simulink model "Case3_Sim"  (R2020b)
settings: Solver=FixedStepAuto  StartTime=0.0  StopTime=10  FixedStep=Ts  RelTol=1e-3
values from neighbouring files (symbols this model uses):
  Cf = 0.02    [Case3_SimPara.m]
  Lc = 1e-9    (= 1e-09)    [Case3_SimPara.m]
  Lf = 0.05    [Case3_SimPara.m]
  Sbase = 1    [Case3_SimPara.m]
  Ts = 1/Fs    (= 0.0001)    [Case3_SimPara.m]
  Vbase = 1    [Case3_SimPara.m]
  w_i = 250*2*pi    (= 1570.79632679)    [Case3_SimPara.m]
  w_pll = 15*2*pi    (= 94.2477796077)    [Case3_SimPara.m]
  w_tau = 1e3*2*pi    (= 6283.18530718)    [Case3_SimPara.m]
  Wbase = 2*pi*50    (= 314.159265359)    [Case3_SimPara.m]
  Ybase = 1/Zbase    (= 1)    [Case3_SimPara.m]
  Zbase = Vbase/Ibase    (= 1)    [Case3_SimPara.m]
undefined symbols (not defined in the file or in its folder): DiscIntNeverNeededParam, initial, m
libraries: SimplexPS x25, powerlib x21
settings Model: Creator=admin_user  LastModifiedBy=admin_user
settings DataIOCC: ReturnWorkspaceOutputs=off

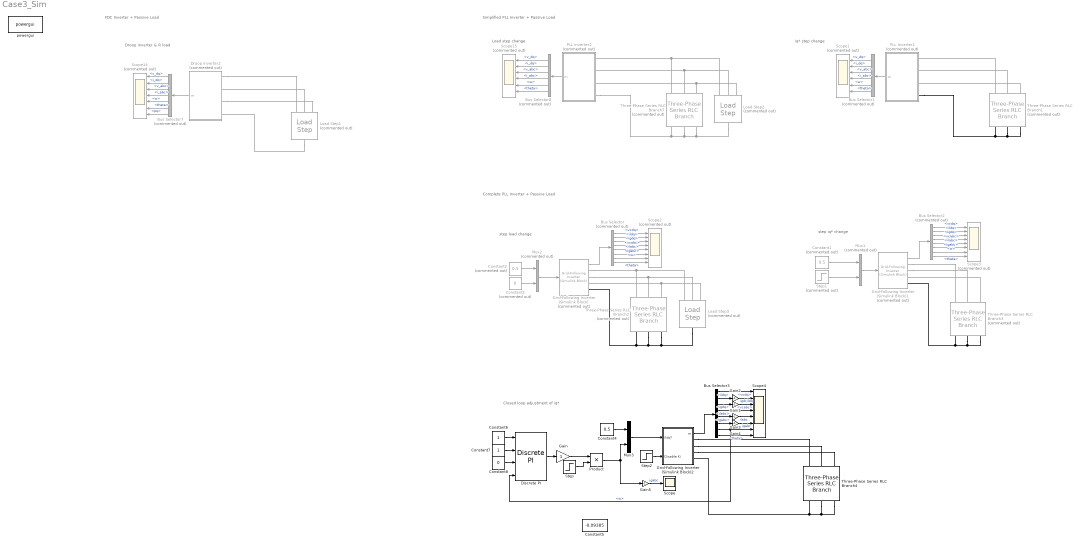
== system Case3_Sim ==
  note: step load change
  note: iq* step change
  note: Load step change
  note: FDC Inverter + Passive Load
  note: Droop inverter & R load
  note: Simplified PLL Inverter + Passive Load
  note: Complete PLL Inverter + Passive Load
  note: step iq* change
  note: Closed loop adjustment of iq*
  Bus Selector : BusSelector  Commented=on  OutputSignals=vcdq,ildq,igdq,vcabc,ilabc,igabc,w,theta
  Bus Selector1 : BusSelector  Commented=on  OutputSignals=v_dq,i_dq,v_abc,i_abc,w,theta
  Bus Selector2 : BusSelector  Commented=on  OutputSignals=vcdq,ildq,igdq,vcabc,ilabc,igabc,w,theta
  Bus Selector3 : BusSelector  OutputSignals=vcdq,ildq,igdq,vcabc,ilabc,igabc,w,theta
  Bus Selector7 : BusSelector  Commented=on  OutputSignals=v_dq,i_dq,v_abc,i_abc,w,theta,pq
  Bus Selector8 : BusSelector  Commented=on  OutputSignals=v_dq,i_dq,v_abc,i_abc,w,theta
  Constant1 : Constant  Commented=on  Value=0.5
  Constant2 : Constant  Commented=on  Value=0.5
  Constant3 : Constant  Commented=on  Value=0
  Constant4 : Constant  Value=0.5
  Constant5 : Constant  Value=-0.09385
  Constant6 : Constant
  Constant7 : Constant
  Constant8 : Constant  Value=0
  Discrete PI : SimplexPS/Discrete PI  Kp=0.5*2*pi/5  Ki=(0.5*2*pi)^2/4/5  xmax=inf  xmin=-inf  Ts=Ts
      settings: SourceProductName=Simplex Power Systems
  Droop Inverter2 : Subsystem  Commented=on
  Gain : Gain
  Gain{1..5} (5 alike) : Gain  Gain=-1
  Grid-Following Inverter (Simulink Block) : SimplexPS/Grid-Following Inverter (Simulink Block)  Commented=on  Ts=Ts  Sbase=Sbase  Vbase=Vbase  Wbase=Wbase  w_i=w_i  w_pll=w_pll  w_tau=w_tau  Lf=Lf  Cf=Cf  Lc=Lc
      link override ControllerAC/Current Controller: Ki=w_i*Lf*w_i/4
      link override Current Controller: Kcd=0
      link override LC Filter: Rd=1e-9
      settings: SourceProductName=Simplex Power Systems
  Grid-Following Inverter (Simulink Block)1 : SimplexPS/Grid-Following Inverter (Simulink Block)  Commented=on  Ts=Ts  Sbase=Sbase  Vbase=Vbase  Wbase=Wbase  w_i=w_i  w_pll=w_pll  w_tau=w_tau  Lf=Lf  Cf=Cf  Lc=Lc
      link override ControllerAC/Current Controller: Ki=w_i*Lf*w_i/4
      link override Current Controller: Kcd=0
      link override LC Filter: Rd=1e-9
      settings: SourceProductName=Simplex Power Systems
  Grid-Following Inverter (Simulink Block)2 : Subsystem  AncestorBlock=|
      | SimplexPS/Grid-Following Inverter
      | (Simulink Block)
  Load Step1 : SimplexPS/Load Step  Commented=on  t0=1  R=2*Zbase  Reverse=0
      settings: SourceProductName=Simplex Power Systems
  Load Step2 : SimplexPS/Load Step  Commented=on  t0=1  R=Zbase  Reverse=0
      settings: SourceProductName=Simplex Power Systems
  Load Step3 : SimplexPS/Load Step  Commented=on  t0=1  R=Zbase  Reverse=0
      settings: SourceProductName=Simplex Power Systems
  Mux1 : Mux  Commented=on  Inputs=2
  Mux2 : Mux  Commented=on  Inputs=2
  Mux3 : Mux  Inputs=2
  PLL Inverter1 : Subsystem  Commented=on
  PLL Inverter2 : Subsystem  Commented=on
  Product : Product
  Scope : Scope
  Scope1 : Scope  Commented=on  NumInputPorts=6
  Scope14 : Scope  Commented=on  NumInputPorts=7
  Scope15 : Scope  Commented=on  NumInputPorts=6
  Scope2 : Scope  Commented=on  NumInputPorts=8
  Scope3 : Scope  Commented=on  NumInputPorts=8
  Scope4 : Scope  NumInputPorts=8
  Step : Step  Time=9  Before=1  After=0  SampleTime=0
  Step1 : Step  Commented=on  After=0.1  SampleTime=0
  Step2 : Step  Time=9.4  Before=1  After=0  SampleTime=0
  Three-Phase Series RLC Branch{1..3,7} (4 alike) : powerlib/Elements/Three-Phase Series RLC Branch  Commented=on  LConnTagsString=A|B|C  RConnTagsString=A|B|C  BranchType=R  Resistance=Zbase  Inductance=0.3*Zbase/Wbase  Capacitance=1/Wbase  Measurements=None
  Three-Phase Series RLC Branch4 : powerlib/Elements/Three-Phase Series RLC Branch  LConnTagsString=A|B|C  RConnTagsString=A|B|C  BranchType=RL  Resistance=Zbase  Inductance=0.2*Zbase/Wbase  Capacitance=1/Wbase  Measurements=None
  powergui : powerlib/powergui  Priority=1  SimulationMode=Discrete  SampleTime=Ts  frequency=60  Iterations=50  frequencyindice=0  Pbase=100e6  ErrMax=1e-4  UnitsV=kV  UnitsW=MW  buscounter=0  FunctionMessages=off  echomessages=off  EnableUseOfTLC=off  CurrentSourceSwitches=off  DisableSnubberDevices=off  DisableRonSwitches=off  DisableVfSwitches=off  DisplayEquations=off  AutomaticDiscreteSolvers=off  SolverType=Tustin/Backward Euler (TBE)  Interpol=off  ExternalGateDelay=off  methode=off  Ts=100  x0status=blocks  SPID=on  SwTol=0  HookPort=off  NonlinearTolerance=1e-4  nMaxIteration=100  ContinueOnMaxIteration=off  RestoreLinks=warning  ResistiveCurrentMeasurement=off  Frange=[0:2:500]  Ylog=off  Xlog=on  ShowGrid=off  save=off  variable=ZData  structure=0  ZoomFFT=off  StartTime=0.0  cycles=1  DisplayStyle=1  fundamental=60  FreqAxis=off  MaxFrequency=1000  frequencyindicesteady=1  RmsSteady=1  display=off
  wires:
  Bus Selector7/3 -> Scope14/3  "<v_abc>"
  Bus Selector7/6 -> Scope14/6  "<theta>"
  Bus Selector7/2 -> Scope14/2  "<i_dq>"
  Bus Selector7/1 -> Scope14/1  "<v_dq>"
  Droop Inverter2/1(m) -> Bus Selector7/1
  Bus Selector7/7 -> Scope14/7  "<pq>"
  Bus Selector7/5 -> Scope14/5  "<w>"
  Bus Selector7/4 -> Scope14/4  "<i_abc>"
  PLL Inverter2/1(m) -> Bus Selector8/1
  Bus Selector8/2 -> Scope15/2  "<i_dq>"
  Bus Selector8/1 -> Scope15/1  "<v_dq>"
  Bus Selector8/4 -> Scope15/4  "<i_abc>"
  Bus Selector8/3 -> Scope15/3  "<v_abc>"
  Bus Selector8/6 -> Scope15/6  "<theta>"
  Bus Selector8/5 -> Scope15/5  "<w>"
  PLL Inverter1/1(m) -> Bus Selector1/1
  Bus Selector1/6 -> Scope1/6  "<theta>"
  Bus Selector1/3 -> Scope1/3  "<v_abc>"
  Bus Selector1/2 -> Scope1/2  "<i_dq>"
  Bus Selector1/1 -> Scope1/1  "<v_dq>"
  Bus Selector1/5 -> Scope1/5  "<w>"
  Bus Selector1/4 -> Scope1/4  "<i_abc>"
  Grid-Following Inverter (Simulink Block)/1 -> Bus Selector/1
  Bus Selector/1 -> Scope2/1  "<vcdq>"
  Bus Selector/2 -> Scope2/2  "<ildq>"
  Bus Selector/3 -> Scope2/3  "<igdq>"
  Bus Selector/4 -> Scope2/4  "<vcabc>"
  Bus Selector/5 -> Scope2/5  "<ilabc>"
  Bus Selector/6 -> Scope2/6  "<igabc>"
  Bus Selector/7 -> Scope2/7  "<w>"
  Bus Selector/8 -> Scope2/8  "<theta>"
  Grid-Following Inverter (Simulink Block)1/1 -> Bus Selector2/1
  Step1/1 -> Mux1/2
  Constant1/1 -> Mux1/1
  Mux1/1 -> Grid-Following Inverter (Simulink Block)1/1
  Bus Selector2/8 -> Scope3/8  "<theta>"
  Bus Selector2/5 -> Scope3/5  "<ilabc>"
  Bus Selector2/7 -> Scope3/7  "<w>"
  Bus Selector2/3 -> Scope3/3  "<igdq>"
  Bus Selector2/4 -> Scope3/4  "<vcabc>"
  Bus Selector2/6 -> Scope3/6  "<igabc>"
  Bus Selector2/1 -> Scope3/1  "<vcdq>"
  Bus Selector2/2 -> Scope3/2  "<ildq>"
  Mux2/1 -> Grid-Following Inverter (Simulink Block)/1
  Constant2/1 -> Mux2/1
  Constant3/1 -> Mux2/2
  Grid-Following Inverter (Simulink Block)2/1(m) -> Bus Selector3/1
  Mux3/1 -> Grid-Following Inverter (Simulink Block)2/1(ildq*)
  Constant4/1 -> Mux3/1
  Bus Selector3/8 -> Scope4/8  "<theta>"
  Bus Selector3/7 -> Discrete PI/4, Scope4/7  "<w>"
  Bus Selector3/4 -> Scope4/4  "<vcabc>"
  Bus Selector3/1 -> Scope4/1  "<vcdq>"
  Constant6/1 -> Discrete PI/1
  Constant7/1 -> Discrete PI/2
  Constant8/1 -> Discrete PI/3
  Product/1 -> Gain5/1, Mux3/2
  Discrete PI/1 -> Gain/1
  Gain/1 -> Product/1
  Step/1 -> Product/2
  Step2/1 -> Grid-Following Inverter (Simulink Block)2/2(Disable Ki)
  Bus Selector3/3 -> Gain1/1  "<igdq>"
  Gain1/1 -> Scope4/3  "igdq"
  Bus Selector3/2 -> Gain2/1  "<ildq>"
  Gain2/1 -> Scope4/2  "ildq"
  Gain3/1 -> Scope4/5  "ilabc"
  Bus Selector3/5 -> Gain3/1  "<ilabc>"
  Gain4/1 -> Scope4/6  "igabc"
  Bus Selector3/6 -> Gain4/1  "<igabc>"
  Gain5/1 -> Scope/1  "igabc"
  connections:
  Droop Inverter2/LConn1 -- Load Step1/LConn1
  Load Step1/LConn2 -- Droop Inverter2/LConn2
  Droop Inverter2/LConn3 -- Load Step1/LConn3
  Load Step1/RConn1 -- Droop Inverter2/LConn4
  Three-Phase Series RLC Branch7/RConn1 -- Load Step2/LConn1 -- PLL Inverter2/LConn1
  Three-Phase Series RLC Branch7/RConn2 -- Load Step2/LConn2 -- PLL Inverter2/LConn2
  Three-Phase Series RLC Branch7/RConn3 -- Load Step2/LConn3 -- PLL Inverter2/LConn3
  PLL Inverter2/LConn4 -- Load Step2/RConn1 -- Three-Phase Series RLC Branch7/LConn3 -- Three-Phase Series RLC Branch7/LConn2 -- Three-Phase Series RLC Branch7/LConn1
  Three-Phase Series RLC Branch1/RConn2 -- PLL Inverter1/LConn2
  Three-Phase Series RLC Branch1/RConn3 -- PLL Inverter1/LConn3
  Three-Phase Series RLC Branch1/LConn1 -- PLL Inverter1/LConn4 -- Three-Phase Series RLC Branch1/LConn3 -- Three-Phase Series RLC Branch1/LConn2
  Three-Phase Series RLC Branch1/RConn1 -- PLL Inverter1/LConn1
  Three-Phase Series RLC Branch2/RConn2 -- Load Step3/LConn2 -- Grid-Following Inverter (Simulink Block)/RConn2
  Three-Phase Series RLC Branch2/RConn3 -- Load Step3/LConn3 -- Grid-Following Inverter (Simulink Block)/RConn3
  Three-Phase Series RLC Branch2/LConn1 -- Load Step3/RConn1 -- Three-Phase Series RLC Branch2/LConn3 -- Three-Phase Series RLC Branch2/LConn2 -- Grid-Following Inverter (Simulink Block)/RConn4
  Load Step3/LConn1 -- Grid-Following Inverter (Simulink Block)/RConn1 -- Three-Phase Series RLC Branch2/RConn1
  Three-Phase Series RLC Branch3/LConn1 -- Grid-Following Inverter (Simulink Block)1/RConn4 -- Three-Phase Series RLC Branch3/LConn3 -- Three-Phase Series RLC Branch3/LConn2
  Three-Phase Series RLC Branch3/RConn3 -- Grid-Following Inverter (Simulink Block)1/RConn3
  Grid-Following Inverter (Simulink Block)1/RConn2 -- Three-Phase Series RLC Branch3/RConn2
  Grid-Following Inverter (Simulink Block)1/RConn1 -- Three-Phase Series RLC Branch3/RConn1
  Three-Phase Series RLC Branch4/LConn1 -- Grid-Following Inverter (Simulink Block)2/RConn4 -- Three-Phase Series RLC Branch4/LConn3 -- Three-Phase Series RLC Branch4/LConn2
  Grid-Following Inverter (Simulink Block)2/RConn2 -- Three-Phase Series RLC Branch4/RConn2
  Grid-Following Inverter (Simulink Block)2/RConn1 -- Three-Phase Series RLC Branch4/RConn1
  Grid-Following Inverter (Simulink Block)2/RConn3 -- Three-Phase Series RLC Branch4/RConn3

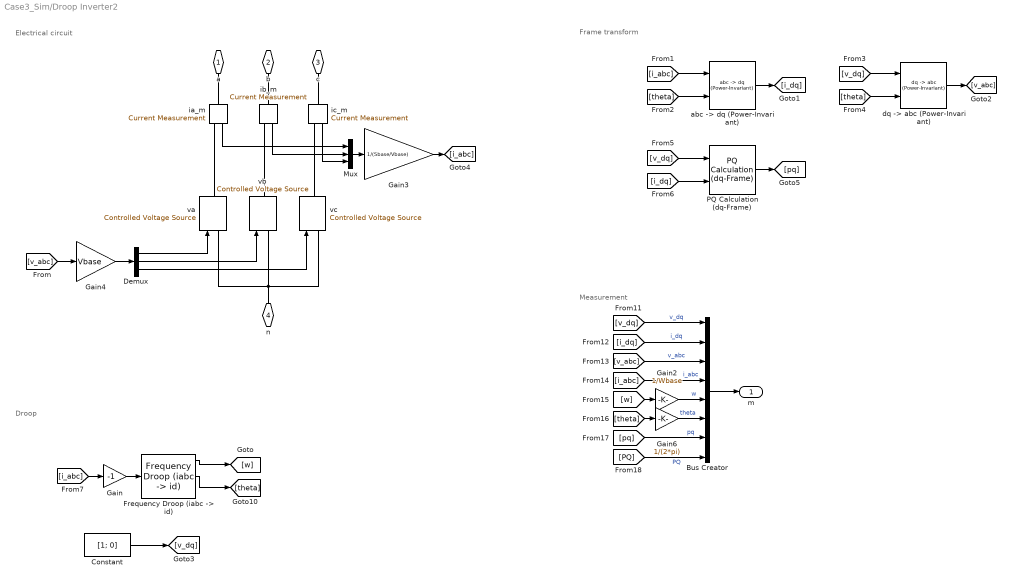
== system Case3_Sim/Droop Inverter2 ==
  note: Measurement
  note: Droop
  note: Frame transform
  note: Electrical circuit
  Bus Creator : BusCreator  Inputs=8
  Constant : Constant  Value=[1; 0]
  Demux : Demux  Outputs=3
  "Frequency Droop (iabc -> id)" : SimplexPS/Frequency Droop (iabc -> id)  Ts=Ts  Sbase=Sbase  Vbase=Vbase  Wbase=Wbase  m=m  w_tau=w_droop  theta0=0  i0=0  w0=1
      settings: SourceProductName=Simplex Power Systems
  Gain : Gain  Gain=-1
  Gain2 : Gain  Gain=1/Wbase
  Gain3 : Gain  Gain=1/(Sbase/Vbase)
  Gain4 : Gain  Gain=Vbase
  Gain6 : Gain  Gain=1/(2*pi)
  Mux : Mux  Inputs=3
  PQ Calculation (dq-Frame) : SimplexPS/PQ Calculation (dq-Frame)  SystemSampleTime=-1  VariantActivationTime=update diagram  Latency=0  AutoFrameSizeCalculation=off
      settings: SourceProductName=Simplex Power Systems
  "abc -> dq (Power-Invariant)" : SimplexPS/abc -> dq (Power-Invariant)  SystemSampleTime=-1  VariantActivationTime=update diagram  Latency=0  AutoFrameSizeCalculation=off
      settings: SourceProductName=Simplex Power Systems
  "dq -> abc (Power-Invariant)" : SimplexPS/dq -> abc (Power-Invariant)  SystemSampleTime=-1  VariantActivationTime=update diagram  Latency=0  AutoFrameSizeCalculation=off
      settings: SourceProductName=Simplex Power Systems
  ia_m : powerlib/Measurements/Current Measurement  PhasorSimulation=off  OutputType=Complex  PSBequivalent=0
  ib_m : powerlib/Measurements/Current Measurement  PhasorSimulation=off  OutputType=Complex  PSBequivalent=0
  ic_m : powerlib/Measurements/Current Measurement  PhasorSimulation=off  OutputType=Complex  PSBequivalent=0
  va : powerlib/Electrical Sources/Controlled Voltage Source  Initialize=on  Source_Type=AC  Amplitude=0  Phase=0  Frequency=0  Measurements=None
  vb : powerlib/Electrical Sources/Controlled Voltage Source  Initialize=on  Source_Type=AC  Amplitude=0  Phase=0  Frequency=0  Measurements=None
  vc : powerlib/Electrical Sources/Controlled Voltage Source  Initialize=on  Source_Type=AC  Amplitude=0  Phase=0  Frequency=0  Measurements=None
  a : PMIOPort  Side=Left
  b : PMIOPort  Port=2  Side=Left
  c : PMIOPort  Port=3  Side=Left
  n : PMIOPort  Port=4  Side=Left
  m : Outport
  wires:
  ic_m/1 -> Mux/3
  ia_m/1 -> Mux/1
  ib_m/1 -> Mux/2
  Demux/1 -> va/1
  Demux/2 -> vb/1
  Demux/3 -> vc/1
  [i_abc] -> "abc -> dq (Power-Invariant)"/1
  [theta] -> "abc -> dq (Power-Invariant)"/2
  "abc -> dq (Power-Invariant)"/1 -> [i_dq]
  [v_dq] -> "dq -> abc (Power-Invariant)"/1
  [theta] -> "dq -> abc (Power-Invariant)"/2
  "dq -> abc (Power-Invariant)"/1 -> [v_abc]
  [v_dq] -> Bus Creator/1  "v_dq"
  [v_abc] -> Bus Creator/3  "v_abc"
  [i_abc] -> Bus Creator/4  "i_abc"
  [pq] -> Bus Creator/7  "pq"
  [PQ] -> Bus Creator/8  "PQ"
  Bus Creator/1 -> m/1
  [w] -> Gain2/1
  Gain2/1 -> Bus Creator/5  "w"
  Mux/1 -> Gain3/1
  Gain3/1 -> [i_abc]
  [v_abc] -> Gain4/1
  Gain4/1 -> Demux/1
  [theta] -> Gain6/1
  Gain6/1 -> Bus Creator/6  "theta"
  "Frequency Droop (iabc -> id)"/2 -> [theta]
  [i_abc] -> Gain/1
  "Frequency Droop (iabc -> id)"/1 -> [w]
  Constant/1 -> [v_dq]
  [i_dq] -> Bus Creator/2  "i_dq"
  [v_dq] -> PQ Calculation (dq-Frame)/1
  [i_dq] -> PQ Calculation (dq-Frame)/2
  PQ Calculation (dq-Frame)/1 -> [pq]
  Gain/1 -> "Frequency Droop (iabc -> id)"/1
  connections:
  ia_m/RConn1 -- va/RConn1
  ia_m/LConn1 -- a/RConn1
  ib_m/RConn1 -- vb/RConn1
  ic_m/RConn1 -- vc/RConn1
  va/LConn1 -- vb/LConn1 -- vc/LConn1 -- n/RConn1
  ib_m/LConn1 -- b/RConn1
  ic_m/LConn1 -- c/RConn1

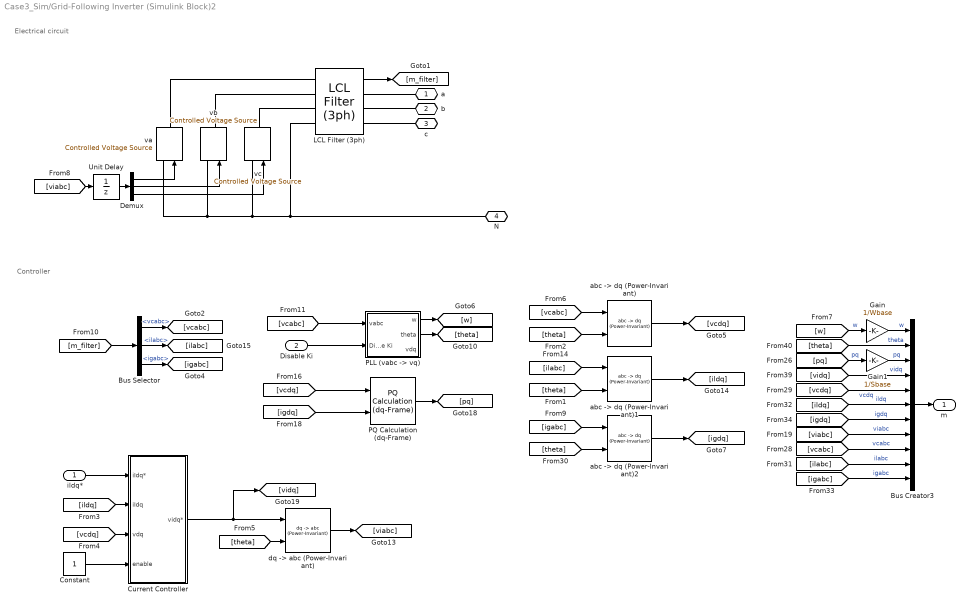
== system Case3_Sim/Grid-Following Inverter (Simulink Block)2 ==
  note: Electrical circuit
  note: Controller
  ildq* : Inport
  Disable Ki : Inport  Port=2
  Bus Creator3 : BusCreator  Inputs=11
  Bus Selector : BusSelector  OutputSignals=vcabc,ilabc,igabc
  Constant : Constant
  Current Controller : Subsystem  mask{Ts=Ts, Wbase=Wbase, Lf=Lf*Zbase/Wbase, Kg=0, Kp=w_i*Lf*Zbase/Wbase, Ki=w_i*w_i/4*Lf*Zbase/Wbase, vdmax=inf, vqmax=inf, Kcd=0}
      mask prompts: Ts "Sampling Time (s)"; Wbase "Base Angular Frequency (rad/s)"; Lf "Inductance"; Kg "Estimator Gain"; Kp "Proportional Gain"; Ki "Integral Gain"; vdmax "Voltage D Limit"; vqmax "Voltage Q Limit"; Kcd "Cross Decoupling Gain"
  Demux : Demux  Outputs=3
  Gain : Gain  Gain=1/Wbase
  Gain1 : Gain  Gain=1/Sbase
  LCL Filter (3ph) : SimplexPS/LCL Filter (3ph)  Lf=Lf*Zbase/Wbase  Rf=Lf/5  Lc=Lc*Zbase/Wbase  Rc=Lc/5  Cf=Cf*Ybase/Wbase  Rd=1e-20
      settings: SourceProductName=Simplex Power System
  "PLL (vabc -> vq)" : Subsystem  AncestorBlock=|  mask{Ts=Ts, Vbase=Vbase, Wbase=Wbase, w_pll=w_pll, w_tau=w_tau, theta0=0}
      | SimplexPS/PLL
      | (vabc -> vq)
      mask prompts: Ts "Ts (s), sampling period"; Vbase "Vbase (V), base voltage"; Wbase "Wbase (rad/s), base angular frequency"; w_pll "w_pll (rad/s), PLL bandwidth"; w_tau "w_tau (rad/s), low-pass filter bandwidth"; theta0 "theta0 (rad), initial angle"
  PQ Calculation (dq-Frame) : SimplexPS/PQ Calculation (dq-Frame)  SystemSampleTime=-1  VariantActivationTime=update diagram  Latency=0  AutoFrameSizeCalculation=off
      settings: SourceProductName=Simplex Power Systems
  Unit Delay : UnitDelay  SampleTime=-1  HasFrameUpgradeWarning=on
  "abc -> dq (Power-Invariant)" : SimplexPS/abc -> dq (Power-Invariant)  SystemSampleTime=-1  VariantActivationTime=update diagram  Latency=0  AutoFrameSizeCalculation=off
      settings: SourceProductName=Simplex Power Systems
  "abc -> dq (Power-Invariant)1" : SimplexPS/abc -> dq (Power-Invariant)  SystemSampleTime=-1  VariantActivationTime=update diagram  Latency=0  AutoFrameSizeCalculation=off
      settings: SourceProductName=Simplex Power Systems
  "abc -> dq (Power-Invariant)2" : SimplexPS/abc -> dq (Power-Invariant)  SystemSampleTime=-1  VariantActivationTime=update diagram  Latency=0  AutoFrameSizeCalculation=off
      settings: SourceProductName=Simplex Power Systems
  "dq -> abc (Power-Invariant)" : SimplexPS/dq -> abc (Power-Invariant)  SystemSampleTime=-1  VariantActivationTime=update diagram  Latency=0  AutoFrameSizeCalculation=off
      settings: SourceProductName=Simplex Power Systems
  va : powerlib/Electrical Sources/Controlled Voltage Source  Initialize=on  Source_Type=AC  Amplitude=0  Phase=0  Frequency=0  Measurements=None
  vb : powerlib/Electrical Sources/Controlled Voltage Source  Initialize=on  Source_Type=AC  Amplitude=0  Phase=0  Frequency=0  Measurements=None
  vc : powerlib/Electrical Sources/Controlled Voltage Source  Initialize=on  Source_Type=AC  Amplitude=0  Phase=0  Frequency=0  Measurements=None
  a : PMIOPort  Side=Right
  b : PMIOPort  Port=2  Side=Right
  c : PMIOPort  Port=3  Side=Right
  N : PMIOPort  Port=4  Side=Right
  m : Outport
  wires:
  [igabc] -> Bus Creator3/11  "igabc"
  [ilabc] -> Bus Creator3/10  "ilabc"
  [vcabc] -> Bus Creator3/9  "vcabc"
  [viabc] -> Bus Creator3/8  "viabc"
  [igdq] -> Bus Creator3/7  "igdq"
  [ildq] -> Bus Creator3/6  "ildq"
  [vcdq] -> Bus Creator3/5  "vcdq"
  [vidq] -> Bus Creator3/4  "vidq"
  Gain1/1 -> Bus Creator3/3  "pq"
  [theta] -> Bus Creator3/2  "theta"
  Gain/1 -> Bus Creator3/1  "w"
  [pq] -> Gain1/1  "pq"
  [w] -> Gain/1  "w"
  Bus Selector/1 -> [vcabc]  "<vcabc>"
  Unit Delay/1 -> Demux/1
  [viabc] -> Unit Delay/1
  [m_filter] -> Bus Selector/1
  "abc -> dq (Power-Invariant)1"/1 -> [ildq]
  "abc -> dq (Power-Invariant)2"/1 -> [igdq]
  "abc -> dq (Power-Invariant)"/1 -> [vcdq]
  [vcabc] -> "PLL (vabc -> vq)"/1(vabc)
  [ildq] -> Current Controller/2(iIdq)
  ildq*/1 -> Current Controller/1(iIdq*)
  [igdq] -> PQ Calculation (dq-Frame)/2
  PQ Calculation (dq-Frame)/1 -> [pq]
  [vcdq] -> PQ Calculation (dq-Frame)/1
  [theta] -> "dq -> abc (Power-Invariant)"/2
  Current Controller/1(vidq*) -> "dq -> abc (Power-Invariant)"/1, [vidq]
  [vcdq] -> Current Controller/3(vdq)
  Constant/1 -> Current Controller/4(enable)
  "PLL (vabc -> vq)"/1(w) -> [w]
  "PLL (vabc -> vq)"/2(theta) -> [theta]
  Bus Selector/2 -> [ilabc]  "<ilabc>"
  Bus Selector/3 -> [igabc]  "<igabc>"
  [theta] -> "abc -> dq (Power-Invariant)2"/2
  [igabc] -> "abc -> dq (Power-Invariant)2"/1
  [ilabc] -> "abc -> dq (Power-Invariant)1"/1
  [vcabc] -> "abc -> dq (Power-Invariant)"/1
  [theta] -> "abc -> dq (Power-Invariant)1"/2
  [theta] -> "abc -> dq (Power-Invariant)"/2
  Demux/3 -> vc/1
  Demux/2 -> vb/1
  Demux/1 -> va/1
  LCL Filter (3ph)/1 -> [m_filter]
  Bus Creator3/1 -> m/1
  "dq -> abc (Power-Invariant)"/1 -> [viabc]
  Disable Ki/1 -> "PLL (vabc -> vq)"/2(Disable Ki)
  connections:
  LCL Filter (3ph)/LConn3 -- vc/RConn1
  N/RConn1 -- LCL Filter (3ph)/LConn4 -- va/LConn1 -- vb/LConn1 -- vc/LConn1
  LCL Filter (3ph)/RConn3 -- c/RConn1
  LCL Filter (3ph)/RConn2 -- b/RConn1
  LCL Filter (3ph)/RConn1 -- a/RConn1
  LCL Filter (3ph)/LConn1 -- va/RConn1
  LCL Filter (3ph)/LConn2 -- vb/RConn1

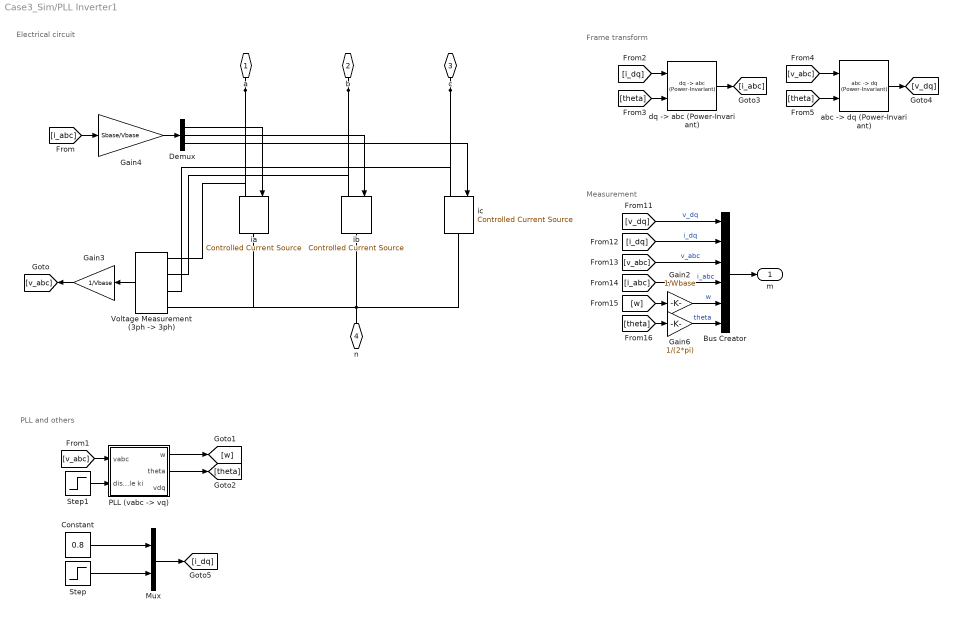
== system Case3_Sim/PLL Inverter1 ==
  note: Measurement
  note: PLL and others
  note: Frame transform
  note: Electrical circuit
  Bus Creator : BusCreator  Inputs=6
  Constant : Constant  Value=0.8
  Demux : Demux  Outputs=3
  Gain2 : Gain  Gain=1/Wbase
  Gain3 : Gain  Gain=1/Vbase
  Gain4 : Gain  Gain=Sbase/Vbase
  Gain6 : Gain  Gain=1/(2*pi)
  Mux : Mux  Inputs=2
  "PLL (vabc -> vq)" : Subsystem  AncestorBlock=|  mask{Ts=Ts, Vbase=Vbase, Wbase=Wbase, w_pll=w_pll, w_tau=w_tau, theta0=0}
      | SimplexPS/PLL
      | (vabc -> vq)
      mask prompts: Ts "Ts (s), sampling period"; Vbase "Vbase (V), base voltage"; Wbase "Wbase (rad/s), base angular frequency"; w_pll "w_pll (rad/s), PLL bandwidth"; w_tau "w_tau (rad/s), low-pass filter bandwidth"; theta0 "theta0 (rad), initial angle"
  Step : Step  Time=0.5  After=0.1  SampleTime=0
  Step1 : Step  Before=1  After=0  SampleTime=Ts
  "Voltage Measurement (3ph -> 3ph)" : SimplexPS/Voltage Measurement (3ph -> 3ph)  SystemSampleTime=-1  VariantActivationTime=update diagram  Latency=0  AutoFrameSizeCalculation=off
      settings: SourceProductName=Simplex Power Systems
  "abc -> dq (Power-Invariant)" : SimplexPS/abc -> dq (Power-Invariant)  SystemSampleTime=-1  VariantActivationTime=update diagram  Latency=0  AutoFrameSizeCalculation=off
      settings: SourceProductName=Simplex Power Systems
  "dq -> abc (Power-Invariant)" : SimplexPS/dq -> abc (Power-Invariant)  SystemSampleTime=-1  VariantActivationTime=update diagram  Latency=0  AutoFrameSizeCalculation=off
      settings: SourceProductName=Simplex Power Systems
  ia : powerlib/Electrical Sources/Controlled Current Source  Initialize=on  Source_Type=AC  Amplitude=0  Phase=0  Frequency=0  Measurements=None
  ib : powerlib/Electrical Sources/Controlled Current Source  Initialize=on  Source_Type=AC  Amplitude=0  Phase=0  Frequency=0  Measurements=None
  ic : powerlib/Electrical Sources/Controlled Current Source  Initialize=on  Source_Type=AC  Amplitude=0  Phase=0  Frequency=0  Measurements=None
  a : PMIOPort  Side=Left
  b : PMIOPort  Port=2  Side=Left
  c : PMIOPort  Port=3  Side=Left
  n : PMIOPort  Port=4  Side=Left
  m : Outport
  wires:
  [v_dq] -> Bus Creator/1  "v_dq"
  [i_dq] -> Bus Creator/2  "i_dq"
  [v_abc] -> Bus Creator/3  "v_abc"
  [i_abc] -> Bus Creator/4  "i_abc"
  Bus Creator/1 -> m/1
  [w] -> Gain2/1
  Gain2/1 -> Bus Creator/5  "w"
  [i_abc] -> Gain4/1
  Gain4/1 -> Demux/1
  [theta] -> Gain6/1
  Gain6/1 -> Bus Creator/6  "theta"
  Demux/1 -> ia/1
  Demux/2 -> ib/1
  Demux/3 -> ic/1
  Gain3/1 -> [v_abc]
  [v_abc] -> "PLL (vabc -> vq)"/1(vabc)
  "PLL (vabc -> vq)"/1(w) -> [w]
  "PLL (vabc -> vq)"/2(theta) -> [theta]
  "Voltage Measurement (3ph -> 3ph)"/1 -> Gain3/1
  "dq -> abc (Power-Invariant)"/1 -> [i_abc]
  [i_dq] -> "dq -> abc (Power-Invariant)"/1
  [theta] -> "dq -> abc (Power-Invariant)"/2
  [v_abc] -> "abc -> dq (Power-Invariant)"/1
  [theta] -> "abc -> dq (Power-Invariant)"/2
  "abc -> dq (Power-Invariant)"/1 -> [v_dq]
  Constant/1 -> Mux/1
  Step/1 -> Mux/2
  Mux/1 -> [i_dq]
  Step1/1 -> "PLL (vabc -> vq)"/2(disable ki)
  connections:
  a/RConn1 -- ia/LConn1 -- "Voltage Measurement (3ph -> 3ph)"/LConn1
  ib/RConn1 -- ic/RConn1 -- n/RConn1 -- ia/RConn1 -- "Voltage Measurement (3ph -> 3ph)"/LConn4
  b/RConn1 -- ib/LConn1 -- "Voltage Measurement (3ph -> 3ph)"/LConn2
  c/RConn1 -- ic/LConn1 -- "Voltage Measurement (3ph -> 3ph)"/LConn3

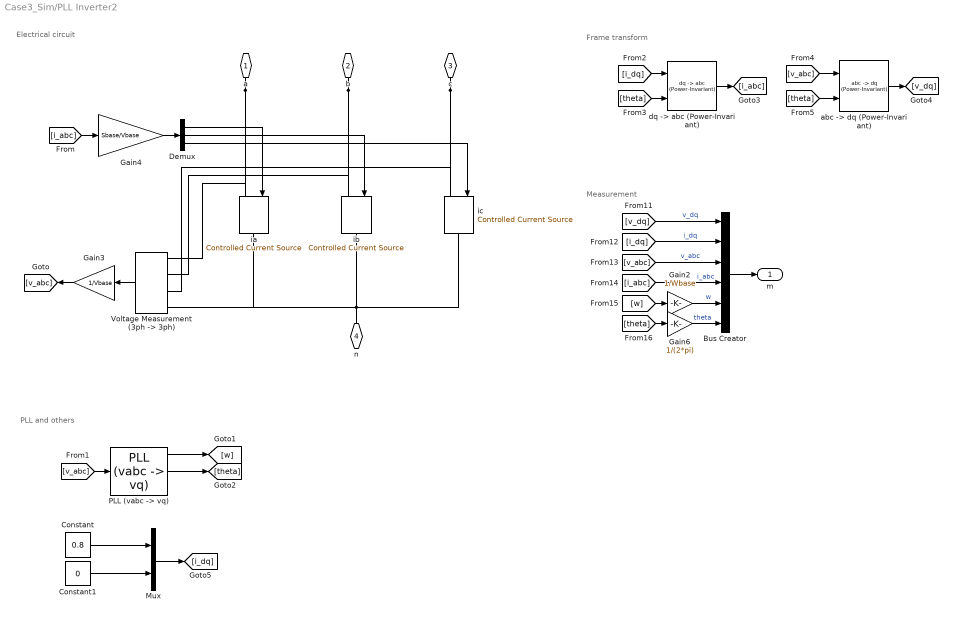
== system Case3_Sim/PLL Inverter2 ==
  note: Measurement
  note: PLL and others
  note: Frame transform
  note: Electrical circuit
  Bus Creator : BusCreator  Inputs=6
  Constant : Constant  Value=0.8
  Constant1 : Constant  Value=0
  Demux : Demux  Outputs=3
  Gain2 : Gain  Gain=1/Wbase
  Gain3 : Gain  Gain=1/Vbase
  Gain4 : Gain  Gain=Sbase/Vbase
  Gain6 : Gain  Gain=1/(2*pi)
  Mux : Mux  Inputs=2
  "PLL (vabc -> vq)" : SimplexPS/PLL (vabc -> vq)  Ts=Ts  Vbase=Vbase  Wbase=Wbase  w_pll=w_pll  w_tau=w_tau  theta0=0
      settings: SourceProductName=Simplex Power Systems
  "Voltage Measurement (3ph -> 3ph)" : SimplexPS/Voltage Measurement (3ph -> 3ph)  SystemSampleTime=-1  VariantActivationTime=update diagram  Latency=0  AutoFrameSizeCalculation=off
      settings: SourceProductName=Simplex Power Systems
  "abc -> dq (Power-Invariant)" : SimplexPS/abc -> dq (Power-Invariant)  SystemSampleTime=-1  VariantActivationTime=update diagram  Latency=0  AutoFrameSizeCalculation=off
      settings: SourceProductName=Simplex Power Systems
  "dq -> abc (Power-Invariant)" : SimplexPS/dq -> abc (Power-Invariant)  SystemSampleTime=-1  VariantActivationTime=update diagram  Latency=0  AutoFrameSizeCalculation=off
      settings: SourceProductName=Simplex Power Systems
  ia : powerlib/Electrical Sources/Controlled Current Source  Initialize=on  Source_Type=AC  Amplitude=0  Phase=0  Frequency=0  Measurements=None
  ib : powerlib/Electrical Sources/Controlled Current Source  Initialize=on  Source_Type=AC  Amplitude=0  Phase=0  Frequency=0  Measurements=None
  ic : powerlib/Electrical Sources/Controlled Current Source  Initialize=on  Source_Type=AC  Amplitude=0  Phase=0  Frequency=0  Measurements=None
  a : PMIOPort  Side=Left
  b : PMIOPort  Port=2  Side=Left
  c : PMIOPort  Port=3  Side=Left
  n : PMIOPort  Port=4  Side=Left
  m : Outport
  wires:
  [v_dq] -> Bus Creator/1  "v_dq"
  [i_dq] -> Bus Creator/2  "i_dq"
  [v_abc] -> Bus Creator/3  "v_abc"
  [i_abc] -> Bus Creator/4  "i_abc"
  Bus Creator/1 -> m/1
  [w] -> Gain2/1
  Gain2/1 -> Bus Creator/5  "w"
  [i_abc] -> Gain4/1
  Gain4/1 -> Demux/1
  [theta] -> Gain6/1
  Gain6/1 -> Bus Creator/6  "theta"
  Demux/1 -> ia/1
  Demux/2 -> ib/1
  Demux/3 -> ic/1
  Gain3/1 -> [v_abc]
  [v_abc] -> "PLL (vabc -> vq)"/1
  "PLL (vabc -> vq)"/1 -> [w]
  "PLL (vabc -> vq)"/2 -> [theta]
  "Voltage Measurement (3ph -> 3ph)"/1 -> Gain3/1
  "dq -> abc (Power-Invariant)"/1 -> [i_abc]
  [i_dq] -> "dq -> abc (Power-Invariant)"/1
  [theta] -> "dq -> abc (Power-Invariant)"/2
  [v_abc] -> "abc -> dq (Power-Invariant)"/1
  [theta] -> "abc -> dq (Power-Invariant)"/2
  "abc -> dq (Power-Invariant)"/1 -> [v_dq]
  Constant/1 -> Mux/1
  Constant1/1 -> Mux/2
  Mux/1 -> [i_dq]
  connections:
  a/RConn1 -- ia/LConn1 -- "Voltage Measurement (3ph -> 3ph)"/LConn1
  ib/RConn1 -- ic/RConn1 -- n/RConn1 -- ia/RConn1 -- "Voltage Measurement (3ph -> 3ph)"/LConn4
  b/RConn1 -- ib/LConn1 -- "Voltage Measurement (3ph -> 3ph)"/LConn2
  c/RConn1 -- ic/LConn1 -- "Voltage Measurement (3ph -> 3ph)"/LConn3

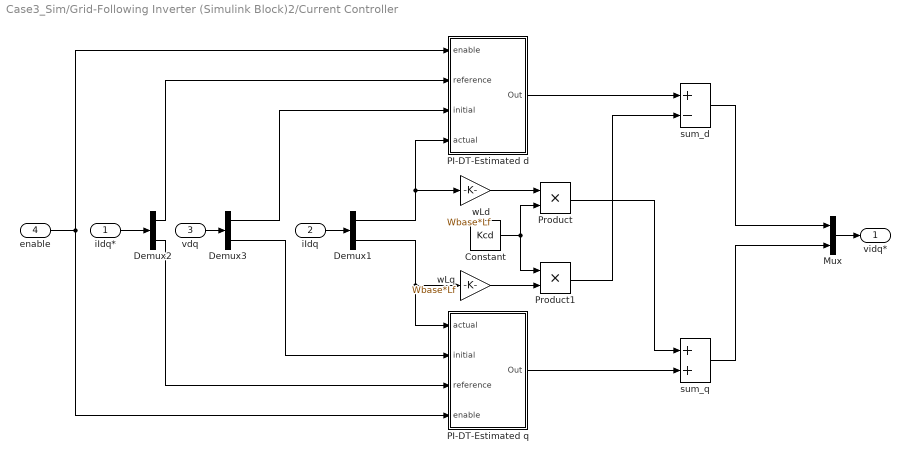
== system Case3_Sim/Grid-Following Inverter (Simulink Block)2/Current Controller ==
  iIdq* : Inport
  iIdq : Inport  Port=2
  vdq : Inport  Port=3
  enable : Inport  Port=4
  Constant : Constant  Value=Kcd
  Demux1 : Demux  Outputs=2
  Demux2 : Demux  Outputs=2
  Demux3 : Demux  Outputs=2
  Mux : Mux  Inputs=2
  PI-DT-Estimated d : Subsystem  mask{Lf=Lf, Kg=Kg, Kp=Kp, Ki=Ki, xmax=vdmax, xmin=-vdmax, Ts=Ts}
      mask prompts: Lf "Inductance"; Kg "Estimator Gain"; Kp "Proportional Gain"; Ki "Integral Gain"; xmax "Upper Limit"; xmin "Lower Limit"; Ts "Sampling Time"
  PI-DT-Estimated q : Subsystem  mask{Lf=Lf, Kg=Kg, Kp=Kp, Ki=Ki, xmax=vqmax, xmin=-vqmax, Ts=Ts}
      mask prompts: Lf "Inductance"; Kg "Estimator Gain"; Kp "Proportional Gain"; Ki "Integral Gain"; xmax "Upper Limit"; xmin "Lower Limit"; Ts "Sampling Time"
  Product : Product
  Product1 : Product
  sum_d : Sum  Inputs=+-
  sum_q : Sum
  wLd : Gain  Gain=Wbase*Lf
  wLq : Gain  Gain=Wbase*Lf
  vidq* : Outport
  wires:
  Constant/1 -> Product1/1, Product/2
  Product1/1 -> sum_d/2
  wLq/1 -> Product1/2
  Product/1 -> sum_q/1
  wLd/1 -> Product/1
  enable/1 -> PI-DT-Estimated d/1(enable), PI-DT-Estimated q/4(enable)
  Demux2/2 -> PI-DT-Estimated q/3(reference)
  Demux2/1 -> PI-DT-Estimated d/2(reference)
  iIdq*/1 -> Demux2/1
  Demux3/1 -> PI-DT-Estimated d/3(initial)
  Demux3/2 -> PI-DT-Estimated q/2(initial)
  PI-DT-Estimated q/1(Out) -> sum_q/2
  vdq/1 -> Demux3/1
  PI-DT-Estimated d/1(Out) -> sum_d/1
  Mux/1 -> vidq*/1
  Demux1/2 -> wLq/1, PI-DT-Estimated q/1(actual)
  Demux1/1 -> PI-DT-Estimated d/4(actual), wLd/1
  iIdq/1 -> Demux1/1
  sum_q/1 -> Mux/2
  sum_d/1 -> Mux/1

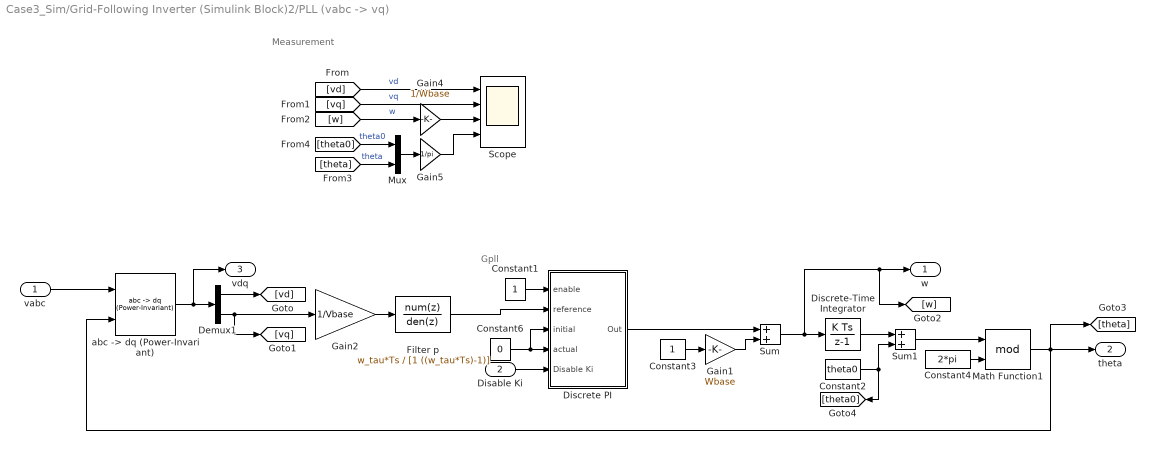
== system Case3_Sim/Grid-Following Inverter (Simulink Block)2/PLL (vabc -> vq) ==
  note: Measurement
  note: Gpll
  vabc : Inport
  Disable Ki : Inport  Port=2
  Constant1 : Constant
  Constant2 : Constant  Value=theta0
  Constant3 : Constant
  Constant4 : Constant  Value=2*pi
  Constant6 : Constant  Value=0
  Demux1 : Demux  Outputs=2
  Discrete PI : Subsystem  AncestorBlock=SimplexPS/Discrete PI  mask{Kp=w_pll, Ki=w_pll*w_pll/4, xmax=inf, xmin=-inf, Ts=Ts}
      mask prompts: Kp "Proportional Gain"; Ki "Integral Gain"; xmax "Upper Limit"; xmin "Lower Limit"; Ts "Sampling Time"
  Discrete-Time Integrator : DiscreteIntegrator  SampleTime=Ts  ICPrevOutput=DiscIntNeverNeededParam  ICPrevScaledInput=DiscIntNeverNeededParam
  Filter p : DiscreteTransferFcn  Numerator=w_tau*Ts  Denominator=[1 ((w_tau*Ts)-1)]  SampleTime=Ts
  Gain1 : Gain  Gain=Wbase
  Gain2 : Gain  Gain=1/Vbase
  Gain4 : Gain  Gain=1/Wbase
  Gain5 : Gain  Gain=1/pi
  Math Function1 : Math  Operator=mod  SignedPower=on  SaturateOnIntegerOverflow=on
  Mux : Mux  Inputs=2
  Scope : Scope  NumInputPorts=4
  Sum : Sum
  Sum1 : Sum
  "abc -> dq (Power-Invariant)" : SimplexPS/abc -> dq (Power-Invariant)  SystemSampleTime=-1  VariantActivationTime=update diagram  Latency=0  AutoFrameSizeCalculation=off
      settings: SourceProductName=Simplex Power Systems
  w : Outport
  theta : Outport  Port=2
  vdq : Outport  Port=3
  wires:
  vabc/1 -> "abc -> dq (Power-Invariant)"/1
  "abc -> dq (Power-Invariant)"/1 -> vdq/1, Demux1/1
  Constant4/1 -> Math Function1/2
  Gain2/1 -> Filter p/1
  Demux1/2 -> [vq], Gain2/1
  Constant6/1 -> Discrete PI/4(actual), Discrete PI/3(initial)
  Constant1/1 -> Discrete PI/1(enable)
  Discrete PI/1(Out) -> Sum/1
  Sum/1 -> [w], w/1, Discrete-Time Integrator/1
  Gain1/1 -> Sum/2
  Discrete-Time Integrator/1 -> Sum1/1
  Sum1/1 -> Math Function1/1
  Constant2/1 -> [theta0], Sum1/2
  Filter p/1 -> Discrete PI/2(reference)
  [vq] -> Scope/2  "vq"
  Mux/1 -> Gain5/1
  Gain4/1 -> Scope/3
  [w] -> Gain4/1  "w"
  [theta0] -> Mux/1  "theta0"
  [vd] -> Scope/1  "vd"
  Gain5/1 -> Scope/4
  [theta] -> Mux/2  "theta"
  Demux1/1 -> [vd]
  Constant3/1 -> Gain1/1
  Math Function1/1 -> "abc -> dq (Power-Invariant)"/2, [theta], theta/1
  Disable Ki/1 -> Discrete PI/5(Disable Ki)

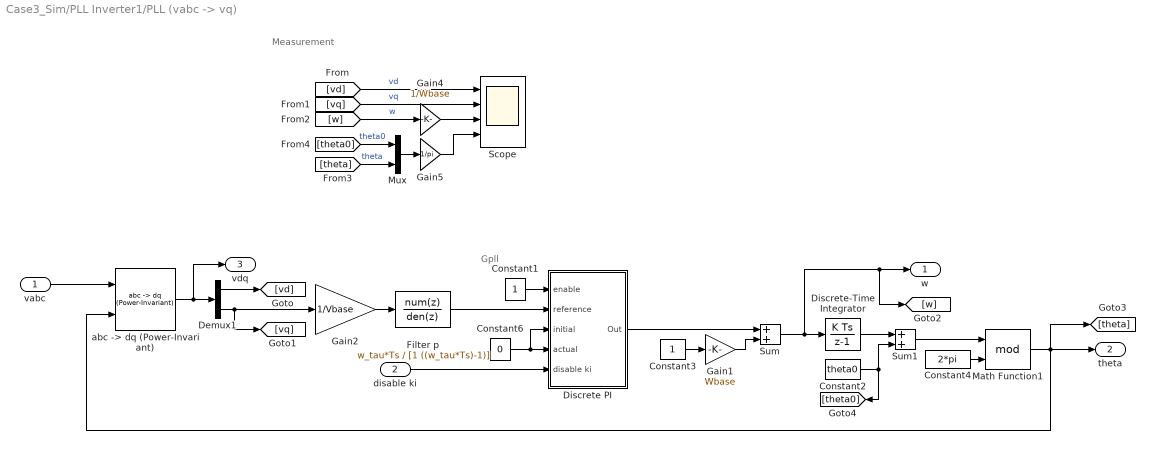
== system Case3_Sim/PLL Inverter1/PLL (vabc -> vq) ==
  note: Measurement
  note: Gpll
  vabc : Inport
  disable ki : Inport  Port=2
  Constant1 : Constant
  Constant2 : Constant  Value=theta0
  Constant3 : Constant
  Constant4 : Constant  Value=2*pi
  Constant6 : Constant  Value=0
  Demux1 : Demux  Outputs=2
  Discrete PI : Subsystem  AncestorBlock=SimplexPS/Discrete PI  mask{Kp=w_pll, Ki=w_pll*w_pll/4, xmax=inf, xmin=-inf, Ts=Ts}
      mask prompts: Kp "Proportional Gain"; Ki "Integral Gain"; xmax "Upper Limit"; xmin "Lower Limit"; Ts "Sampling Time"
  Discrete-Time Integrator : DiscreteIntegrator  SampleTime=Ts  ICPrevOutput=DiscIntNeverNeededParam  ICPrevScaledInput=DiscIntNeverNeededParam
  Filter p : DiscreteTransferFcn  Numerator=w_tau*Ts  Denominator=[1 ((w_tau*Ts)-1)]  SampleTime=Ts
  Gain1 : Gain  Gain=Wbase
  Gain2 : Gain  Gain=1/Vbase
  Gain4 : Gain  Gain=1/Wbase
  Gain5 : Gain  Gain=1/pi
  Math Function1 : Math  Operator=mod  SignedPower=on  SaturateOnIntegerOverflow=on
  Mux : Mux  Inputs=2
  Scope : Scope  NumInputPorts=4
  Sum : Sum
  Sum1 : Sum
  "abc -> dq (Power-Invariant)" : SimplexPS/abc -> dq (Power-Invariant)  SystemSampleTime=-1  VariantActivationTime=update diagram  Latency=0  AutoFrameSizeCalculation=off
      settings: SourceProductName=Simplex Power Systems
  w : Outport
  theta : Outport  Port=2
  vdq : Outport  Port=3
  wires:
  vabc/1 -> "abc -> dq (Power-Invariant)"/1
  "abc -> dq (Power-Invariant)"/1 -> vdq/1, Demux1/1
  Constant4/1 -> Math Function1/2
  Gain2/1 -> Filter p/1
  Demux1/2 -> [vq], Gain2/1
  Constant6/1 -> Discrete PI/4(actual), Discrete PI/3(initial)
  Constant1/1 -> Discrete PI/1(enable)
  Discrete PI/1(Out) -> Sum/1
  Sum/1 -> [w], w/1, Discrete-Time Integrator/1
  Gain1/1 -> Sum/2
  Discrete-Time Integrator/1 -> Sum1/1
  Sum1/1 -> Math Function1/1
  Constant2/1 -> [theta0], Sum1/2
  Filter p/1 -> Discrete PI/2(reference)
  [vq] -> Scope/2  "vq"
  Mux/1 -> Gain5/1
  Gain4/1 -> Scope/3
  [w] -> Gain4/1  "w"
  [theta0] -> Mux/1  "theta0"
  [vd] -> Scope/1  "vd"
  Gain5/1 -> Scope/4
  [theta] -> Mux/2  "theta"
  Demux1/1 -> [vd]
  Constant3/1 -> Gain1/1
  Math Function1/1 -> "abc -> dq (Power-Invariant)"/2, [theta], theta/1
  disable ki/1 -> Discrete PI/5(disable ki)

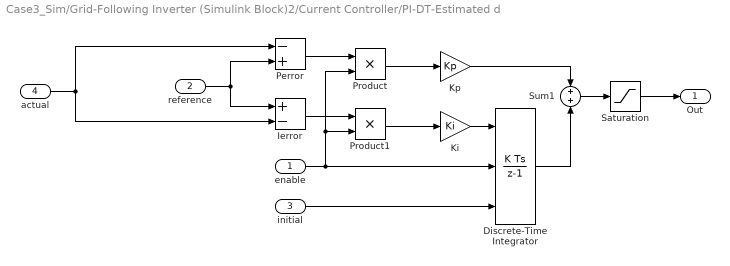
== system Case3_Sim/Grid-Following Inverter (Simulink Block)2/Current Controller/PI-DT-Estimated d ==
  enable : Inport
  reference : Inport  Port=2
  initial : Inport  Port=3
  actual : Inport  Port=4
  Discrete-Time Integrator : DiscreteIntegrator  gainval=1  ExternalReset=rising  InitialConditionSource=external  InitialCondition=initial  SampleTime=Ts  LimitOutput=on  UpperSaturationLimit=xmax  LowerSaturationLimit=xmin  ICPrevOutput=DiscIntNeverNeededParam  ICPrevScaledInput=DiscIntNeverNeededParam
  Ierror : Sum  Inputs=+-
  Ki : Gain  Gain=Ki  SaturateOnIntegerOverflow=on  OutDataTypeStr=Inherit: Same as input  ParamDataTypeStr=Inherit: Same as input
  Kp : Gain  Gain=Kp  SaturateOnIntegerOverflow=on  OutDataTypeStr=Inherit: Same as input  ParamDataTypeStr=Inherit: Same as input
  Perror : Sum  Inputs=-+
  Product : Product  RndMeth=Zero
  Product1 : Product  RndMeth=Zero
  Saturation : Saturate  UpperLimit=xmax  LowerLimit=xmin
  Sum1 : Sum  SaturateOnIntegerOverflow=on
  Out : Outport
  wires:
  Product1/1 -> Ki/1
  Ierror/1 -> Product1/1
  Product/1 -> Kp/1
  Perror/1 -> Product/1
  reference/1 -> Ierror/1, Perror/2
  actual/1 -> Ierror/2, Perror/1
  initial/1 -> Discrete-Time Integrator/3
  enable/1 -> Product1/2, Product/2, Discrete-Time Integrator/2
  Discrete-Time Integrator/1 -> Sum1/2
  Kp/1 -> Sum1/1
  Ki/1 -> Discrete-Time Integrator/1
  Sum1/1 -> Saturation/1
  Saturation/1 -> Out/1

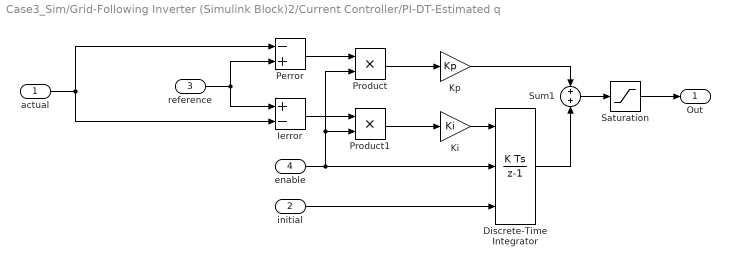
== system Case3_Sim/Grid-Following Inverter (Simulink Block)2/Current Controller/PI-DT-Estimated q ==
  actual : Inport
  initial : Inport  Port=2
  reference : Inport  Port=3
  enable : Inport  Port=4
  Discrete-Time Integrator : DiscreteIntegrator  gainval=1  ExternalReset=rising  InitialConditionSource=external  InitialCondition=initial  SampleTime=Ts  LimitOutput=on  UpperSaturationLimit=xmax  LowerSaturationLimit=xmin  ICPrevOutput=DiscIntNeverNeededParam  ICPrevScaledInput=DiscIntNeverNeededParam
  Ierror : Sum  Inputs=+-
  Ki : Gain  Gain=Ki  SaturateOnIntegerOverflow=on  OutDataTypeStr=Inherit: Same as input  ParamDataTypeStr=Inherit: Same as input
  Kp : Gain  Gain=Kp  SaturateOnIntegerOverflow=on  OutDataTypeStr=Inherit: Same as input  ParamDataTypeStr=Inherit: Same as input
  Perror : Sum  Inputs=-+
  Product : Product  RndMeth=Zero
  Product1 : Product  RndMeth=Zero
  Saturation : Saturate  UpperLimit=xmax  LowerLimit=xmin
  Sum1 : Sum  SaturateOnIntegerOverflow=on
  Out : Outport
  wires:
  Product1/1 -> Ki/1
  Ierror/1 -> Product1/1
  Product/1 -> Kp/1
  Perror/1 -> Product/1
  reference/1 -> Ierror/1, Perror/2
  actual/1 -> Perror/1, Ierror/2
  initial/1 -> Discrete-Time Integrator/3
  enable/1 -> Product1/2, Product/2, Discrete-Time Integrator/2
  Discrete-Time Integrator/1 -> Sum1/2
  Kp/1 -> Sum1/1
  Ki/1 -> Discrete-Time Integrator/1
  Sum1/1 -> Saturation/1
  Saturation/1 -> Out/1

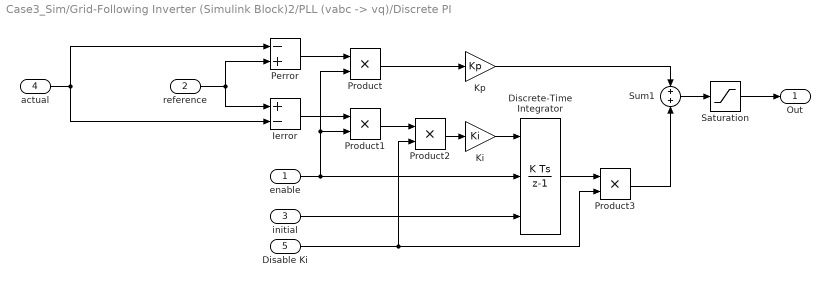
== system Case3_Sim/Grid-Following Inverter (Simulink Block)2/PLL (vabc -> vq)/Discrete PI ==
  enable : Inport
  reference : Inport  Port=2
  initial : Inport  Port=3
  actual : Inport  Port=4
  Disable Ki : Inport  Port=5
  Discrete-Time Integrator : DiscreteIntegrator  gainval=1  ExternalReset=rising  InitialConditionSource=external  InitialCondition=initial  SampleTime=Ts  LimitOutput=on  UpperSaturationLimit=xmax  LowerSaturationLimit=xmin  ICPrevOutput=DiscIntNeverNeededParam  ICPrevScaledInput=DiscIntNeverNeededParam
  Ierror : Sum  Inputs=+-
  Ki : Gain  Gain=Ki  SaturateOnIntegerOverflow=on  OutDataTypeStr=Inherit: Same as input  ParamDataTypeStr=Inherit: Same as input
  Kp : Gain  Gain=Kp  SaturateOnIntegerOverflow=on  OutDataTypeStr=Inherit: Same as input  ParamDataTypeStr=Inherit: Same as input
  Perror : Sum  Inputs=-+
  Product : Product  RndMeth=Zero
  Product1 : Product  RndMeth=Zero
  Product2 : Product
  Product3 : Product
  Saturation : Saturate  UpperLimit=xmax  LowerLimit=xmin
  Sum1 : Sum  SaturateOnIntegerOverflow=on
  Out : Outport
  wires:
  Ierror/1 -> Product1/1
  Product/1 -> Kp/1
  Perror/1 -> Product/1
  actual/1 -> Perror/1, Ierror/2
  reference/1 -> Ierror/1, Perror/2
  initial/1 -> Discrete-Time Integrator/3
  enable/1 -> Product1/2, Product/2, Discrete-Time Integrator/2
  Kp/1 -> Sum1/1
  Ki/1 -> Discrete-Time Integrator/1
  Sum1/1 -> Saturation/1
  Saturation/1 -> Out/1
  Product2/1 -> Ki/1
  Product1/1 -> Product2/1
  Disable Ki/1 -> Product3/2, Product2/2
  Discrete-Time Integrator/1 -> Product3/1
  Product3/1 -> Sum1/2

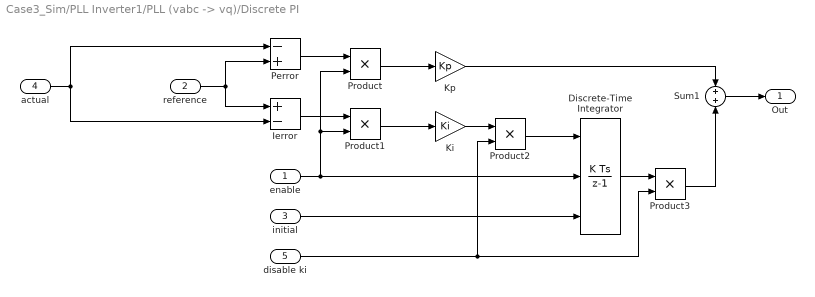
== system Case3_Sim/PLL Inverter1/PLL (vabc -> vq)/Discrete PI ==
  enable : Inport
  reference : Inport  Port=2
  initial : Inport  Port=3
  actual : Inport  Port=4
  disable ki : Inport  Port=5
  Discrete-Time Integrator : DiscreteIntegrator  gainval=1  ExternalReset=rising  InitialConditionSource=external  InitialCondition=initial  SampleTime=Ts  UpperSaturationLimit=xmax  LowerSaturationLimit=xmin  ICPrevOutput=DiscIntNeverNeededParam  ICPrevScaledInput=DiscIntNeverNeededParam
  Ierror : Sum  Inputs=+-
  Ki : Gain  Gain=Ki  SaturateOnIntegerOverflow=on  OutDataTypeStr=Inherit: Same as input  ParamDataTypeStr=Inherit: Same as input
  Kp : Gain  Gain=Kp  SaturateOnIntegerOverflow=on  OutDataTypeStr=Inherit: Same as input  ParamDataTypeStr=Inherit: Same as input
  Perror : Sum  Inputs=-+
  Product : Product  RndMeth=Zero
  Product1 : Product  RndMeth=Zero
  Product2 : Product
  Product3 : Product
  Sum1 : Sum  SaturateOnIntegerOverflow=on
  Out : Outport
  wires:
  Product1/1 -> Ki/1
  Ierror/1 -> Product1/1
  Product/1 -> Kp/1
  Perror/1 -> Product/1
  actual/1 -> Perror/1, Ierror/2
  reference/1 -> Ierror/1, Perror/2
  initial/1 -> Discrete-Time Integrator/3
  enable/1 -> Product1/2, Product/2, Discrete-Time Integrator/2
  Kp/1 -> Sum1/1
  Sum1/1 -> Out/1
  Ki/1 -> Product2/1
  Product2/1 -> Discrete-Time Integrator/1
  Discrete-Time Integrator/1 -> Product3/1
  Product3/1 -> Sum1/2
  disable ki/1 -> Product2/2, Product3/2
